simulink model "testing"  (R2024a)
settings: Solver=FixedStepAuto  StartTime=0.0  StopTime=10  FixedStep=0.0001  RelTol=1e-3
values from neighbouring files (symbols this model uses):
  A = [ 0,      1 ... (first row only)    [simpl_RLC_model.m]
  B = [   0 ... (first row only)    [simpl_RLC_model.m]
  C = [1, 0]    [simpl_RLC_model.m]
  D = [0]    [simpl_RLC_model.m]
settings Model: Creator=jedua  LastModifiedBy=jedua
settings SolverCC: AlgebraicLoopSolver=TrustRegion
settings DebuggingCC: UnconnectedInputMsg=warning  UnconnectedOutputMsg=warning  UnconnectedLineMsg=warning
settings ModelReferenceCC: EnableRefExpFcnMdlSchedulingChecks=on
settings RTWCC: GPUComputeCapability=3.5

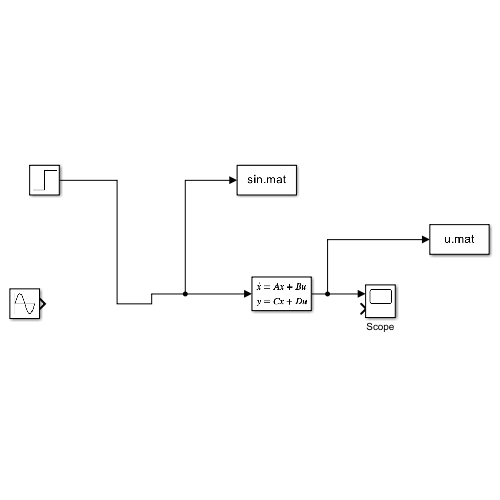
[thumbnail: Simulink's stored preview of the top-level diagram]
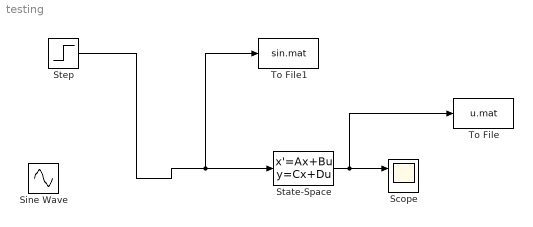
== system testing ==
  Scope : Scope  NumInputPorts=2
  Sine Wave : Sin  Amplitude=100  Frequency=10  SampleTime=0
  State-Space : StateSpace  A=A  B=B  C=C  D=D  InitialCondition=0
  Step : Step  Time=0  After=100  SampleTime=0
  To File : ToFile  Filename=u.mat  MatrixName=u
  To File1 : ToFile  Filename=sin.mat  MatrixName=sin
  wires:
  State-Space/1 -> To File/1, Scope/1
  Step/1 -> To File1/1, State-Space/1
